simulink model "openloopmodel_saturationb_control101"  (R2025b)
settings: Solver=VariableStepAuto  StartTime=0.0  StopTime=stoptime  RelTol=1e-3
undefined symbols (not defined in the file or in its folder): den, gain, num, target, umax, umin
settings Model: Creator=Anthony Rossiter  LastModifiedBy=Anthony Rossiter

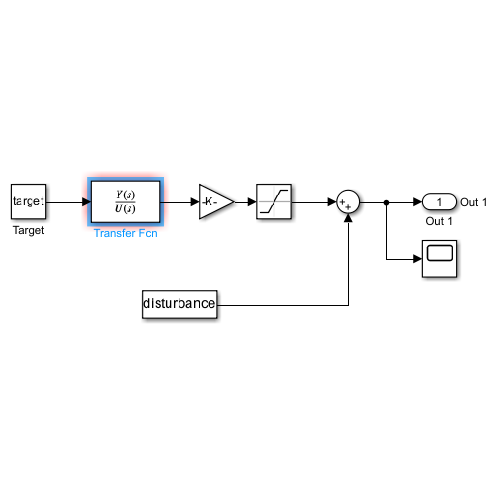
[thumbnail: Simulink's stored preview of the top-level diagram]
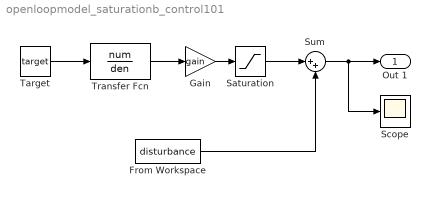
== system openloopmodel_saturationb_control101 ==
  From Workspace : FromWorkspace  VariableName=disturbance
  Gain : Gain  Gain=gain
  Saturation : Saturate  UpperLimit=umax  LowerLimit=umin
  Scope : Scope
  Sum : Sum  Inputs=|++
  Target : Constant  Value=target
  Transfer Fcn : TransferFcn  Numerator=num  Denominator=den
  Out 1 : Outport  SignalName=Out 1
  wires:
  Target/1 -> Transfer Fcn/1
  Gain/1 -> Saturation/1
  Transfer Fcn/1 -> Gain/1
  Saturation/1 -> Sum/1
  Sum/1 -> Scope/1, Out 1/1
  From Workspace/1 -> Sum/2
